simulink model "ac_reciprocal"  (Simulink 9.0)
settings: Solver=FixedStepAuto  StartTime=0.0  StopTime=10  FixedStep=0.001  RelTol=1e-3
libraries: simulink x1, catapult_blocks_lib x1
settings Model: SuppressorTable=22 serialization::archive 11 0 6 0 0 0 11 0  Creator=kharer  LastModifiedBy=kharer
settings DataIOCC: SaveFormat=Dataset
settings OptimizationCC: LifeSpan=auto
settings DebuggingCC: UnderspecifiedInitializationDetection=Simplified  MergeDetectMultiDrivingBlocksExec=error  SFUnexpectedBacktrackingDiag=error  SFNoUnconditionalDefaultTransitionDiag=error  SFExecutionAtInitializationDiag=warning
settings HardwareCC: ProdBitPerPointer=64  ProdBitPerSizeT=64  ProdBitPerPtrDiffT=64  ProdLargestAtomicFloat=Float  ProdIntDivRoundTo=Zero  ProdEndianess=LittleEndian  ProdWordSize=64  ProdHWDeviceType=Intel->x86-64 (Windows64)
settings ModelReferenceCC: PropagateSignalLabelsOutOfModel=on
settings CodeAppCC: StateflowObjectComments=off
settings GRTTargetCC: TargetLangStandard=C99 (ISO)
settings ConfigComp: CovMetricSettings=dwe  CovHtmlReporting=off  CovSaveCumulativeToWorkspaceVar=off  CovSaveSingleToWorkspaceVar=off  CovExternalEMLEnable=on

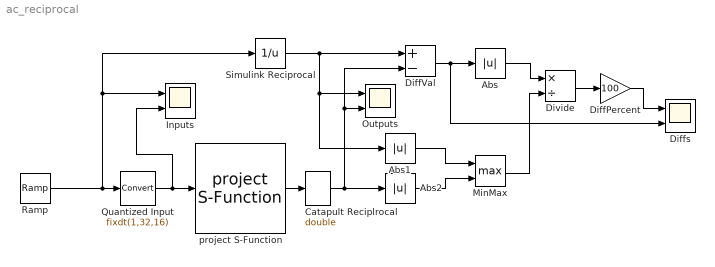
== system ac_reciprocal ==
  Abs : Abs
  Abs1 : Abs
  Abs2 : Abs
  Catapult Reciplrocal : DataTypeConversion  OutDataTypeStr=double  RndMeth=Round  SaturateOnIntegerOverflow=on
  DiffPercent : Gain  Gain=100
  DiffVal : Sum  Inputs=+-
  Diffs : Scope  NumInputPorts=2
  Divide : Product  Inputs=*/
  Inputs : Scope  NumInputPorts=2
  MinMax : MinMax  Function=max  Inputs=2
  Outputs : Scope  NumInputPorts=2
  Quantized Input : DataTypeConversion  OutDataTypeStr=fixdt(1,32,16)  RndMeth=Round  SaturateOnIntegerOverflow=on
  Ramp : simulink/Sources/Ramp  slope=3  start=0  X0=-15
  Simulink Reciprocal : Math  Operator=reciprocal  SaturateOnIntegerOverflow=on
  project S-Function : catapult_blocks_lib/project S-Function  Description=|
      | Description S-Function wrapper around the Catapult C++ function 'project'.
      | Catapult project file: '/wv/fv_engr/kevin/space/ac_reciprocal/Catapult.ccs'
  wires:
  Quantized Input/1 -> Inputs/2, project S-Function/1
  Catapult Reciplrocal/1 -> Abs2/1, DiffVal/2, Outputs/2
  project S-Function/1 -> Catapult Reciplrocal/1
  Ramp/1 -> Simulink Reciprocal/1, Inputs/1, Quantized Input/1
  Simulink Reciprocal/1 -> Abs1/1, Outputs/1, DiffVal/1
  Abs/1 -> Divide/1
  Divide/1 -> DiffPercent/1
  DiffPercent/1 -> Diffs/1
  DiffVal/1 -> Diffs/2, Abs/1
  Abs1/1 -> MinMax/1
  Abs2/1 -> MinMax/2
  MinMax/1 -> Divide/2
